simulink model "JCA_LC_Network_Simulation_0p05_Lambda_In_211003"  (R2020a)
settings: Solver=ode15s  StartTime=0.0  StopTime=100*Td  MaxStep=Td/1000  RelTol=1e-3  EnableMultiTasking=on
PreLoadFcn:
  | load gauss_fir;  % pulse shaping coefficients
InitFcn:
  | Zo   =   50;                 %  Line Impedance
  | 
  | Td   =   1/10e6;              % Sinewave period
  | 
  | Ts   =    Td/50     % set this to control simulation speed
  |                           % for wave visualization
  | Tg   =    Td/500;
  | 
  | N=50;                           % secondary to primary turns ratio
  | Cpl_dB=-20*log10(N);    % Coupler coupling coefficent (dB)
libraries: fl_lib x28, nesl_utility x11, simulink x3, ee_lib x2
settings Model: Creator=Dick  LastModifiedBy=Jeff
settings DataIOCC: LimitDataPoints=on  SaveFormat=Array  ReturnWorkspaceOutputs=off
settings OptimizationCC: LifeSpan=inf
settings DebuggingCC: SolverPrmCheckMsg=warning  SFUnexpectedBacktrackingDiag=warning  SFNoUnconditionalDefaultTransitionDiag=warning  SFExecutionAtInitializationDiag=none  ArithmeticOperatorsInVariantConditions=warning
settings HardwareCC: ProdBitPerPointer=32  ProdBitPerSizeT=32  ProdBitPerPtrDiffT=32  ProdLargestAtomicFloat=None  ProdIntDivRoundTo=Undefined  ProdEndianess=Unspecified  ProdWordSize=32  ProdHWDeviceType=32-bit Generic
settings ModelReferenceCC: PropagateSignalLabelsOutOfModel=off
settings SFSimCC: SimUseLocalCustomCode=off  CustomCodeUndefinedFunction=UseInterfaceOnly
settings RTWCC: RTWUseLocalCustomCode=off
settings CodeAppCC: StateflowObjectComments=on
settings GRTTargetCC: TargetLangStandard=C89/C90 (ANSI)
settings ConfigComp: CovMetricSettings=dw  CovHtmlReporting=on  CovSaveCumulativeToWorkspaceVar=on  CovSaveSingleToWorkspaceVar=on  CovExternalEMLEnable=off  CovSFcnEnable=off
settings SimscapeCC: SimscapeNormalizeSystem=off

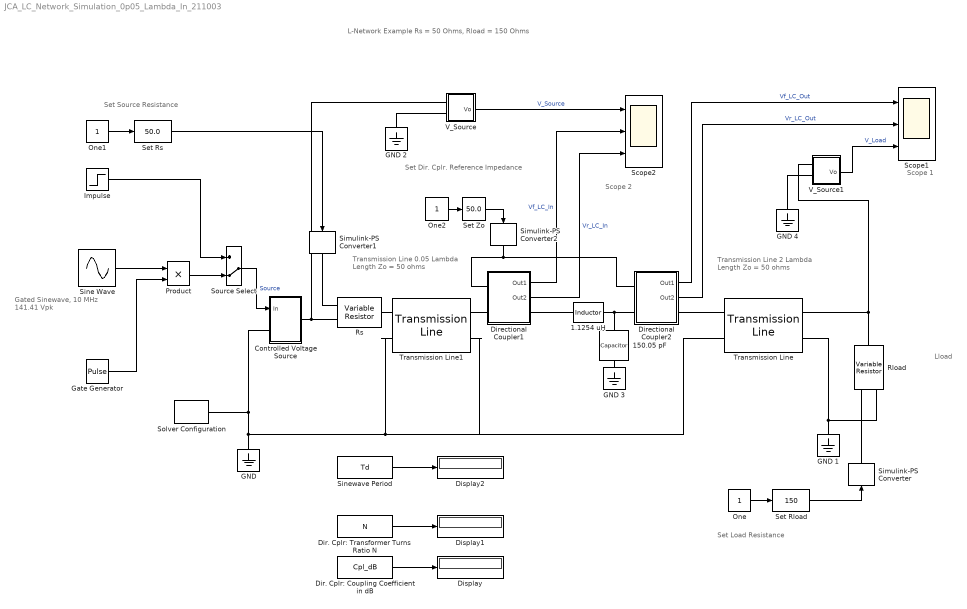
== system JCA_LC_Network_Simulation_0p05_Lambda_In_211003 ==
  note: Lload
  note: Scope 1
  note: L-Network Example
      | Rs = 50 Ohms, Rload = 150 Ohms
  note: Set Load Resistance
  note: Set Source Resistance
  note: Set Dir. Cplr.
      | Reference Impedance
  note: Gated Sinewave,
      | 10 MHz
      | 141.41 Vpk
  note: Transmission Line
      | 2 Lambda Length
      | Zo = 50 ohms
  note: Transmission Line
      | 0.05 Lambda Length
      | Zo = 50 ohms
  note: Scope 2
  1.1254 uH : fl_lib/Electrical/Electrical Elements/Inductor  l=1.1254 uH  r=0 Ohm  g=1e-9 1/Ohm  i_specify=off  i_priority=None  i=0 A  i_nominal_specify=off  i_nominal_unit=A  i_nominal_value=1  v_specify=off  v_priority=None  v=0 V  v_nominal_specify=off  v_nominal_unit=V  v_nominal_value=1  i_L_specify=off  i_L_priority=High  i_L=0 A  i_L_nominal_specify=off  i_L_nominal_unit=A  i_L_nominal_value=1
  150.05 pF : fl_lib/Electrical/Electrical Elements/Capacitor  c=150.05 pF  r=1e-6 Ohm  g=0 1/Ohm  i_specify=off  i_priority=None  i=0 A  i_nominal_specify=off  i_nominal_unit=A  i_nominal_value=1  v_specify=off  v_priority=None  v=0 V  v_nominal_specify=off  v_nominal_unit=V  v_nominal_value=1  vc_specify=off  vc_priority=High  vc=0 V  vc_nominal_specify=off  vc_nominal_unit=V  vc_nominal_value=1
  Controlled Voltage Source : Subsystem
  Dir. Cplr: Coupling Coefficient in dB : Constant  Value=Cpl_dB
  Dir. Cplr: Transformer Turns Ratio N : Constant  Value=N
  Directional Coupler1 : Subsystem
  Directional Coupler2 : Subsystem
  Display : Display
  Display1 : Display
  Display2 : Display
  GND {,1..4} (5 alike) : fl_lib/Electrical/Electrical Elements/Electrical Reference
  Gate Generator : DiscretePulseGenerator  PulseType=Time based  Period=100*Td  PulseWidth=50
  Impulse : Step  Time=Td/1e6  Before=1e13  After=0  SampleTime=0
  One : Constant
  One1 : Constant
  One2 : Constant
  Product : Product
  Rload : fl_lib/Electrical/Electrical Elements/Variable Resistor  Rmin=0 Ohm  i_specify=off  i_priority=High  i=0 A  i_nominal_specify=off  i_nominal_unit=A  i_nominal_value=1  v_specify=off  v_priority=High  v=0 V  v_nominal_specify=off  v_nominal_unit=V  v_nominal_value=1
  Rs : fl_lib/Electrical/Electrical Elements/Variable Resistor  Rmin=0 Ohm  i_specify=off  i_priority=High  i=0 A  i_nominal_specify=off  i_nominal_unit=A  i_nominal_value=1  v_specify=off  v_priority=High  v=0 V  v_nominal_specify=off  v_nominal_unit=V  v_nominal_value=1
  Scope1 : Scope  NumInputPorts=3
  Scope2 : Scope  NumInputPorts=3
  Set Rload : simulink/Math Operations/Slider Gain  gain=150  low=0  high=500
  Set Rs : simulink/Math Operations/Slider Gain  gain=50.0  low=0  high=500
  Set Zo : simulink/Math Operations/Slider Gain  gain=50.0  low=0  high=500
  Simulink-PS Converter : nesl_utility/Simulink-PS Converter  PhysicalDomain=network_engine_domain  SubClassName=ps_input  LeftPortType=input  RightPortType=output  PseudoPeriodic=off  Frequencies=[]  NoiseDistribution=none  NoiseParameters=[]  Unit=1  AffineConversion=off  FilteringAndDerivatives=zero  SimscapeFilterOrder=1  InputFilterTimeConstant=0.001  UdotUserProvided=1
  Simulink-PS Converter1 : nesl_utility/Simulink-PS Converter  PhysicalDomain=network_engine_domain  SubClassName=ps_input  LeftPortType=input  RightPortType=output  PseudoPeriodic=off  Frequencies=[]  NoiseDistribution=none  NoiseParameters=[]  Unit=1  AffineConversion=off  FilteringAndDerivatives=zero  SimscapeFilterOrder=1  InputFilterTimeConstant=0.001  UdotUserProvided=1
  Simulink-PS Converter2 : nesl_utility/Simulink-PS Converter  PhysicalDomain=network_engine_domain  SubClassName=ps_input  LeftPortType=input  RightPortType=output  PseudoPeriodic=off  Frequencies=[]  NoiseDistribution=none  NoiseParameters=[]  Unit=1  AffineConversion=off  FilteringAndDerivatives=zero  SimscapeFilterOrder=1  InputFilterTimeConstant=0.001  UdotUserProvided=1
  Sine Wave : Sin  Amplitude=141.41  Frequency=2*pi/Td  Samples=500  SampleTime=0
  Sinewave Period : Constant  Value=Td
  Solver Configuration : nesl_utility/Solver Configuration  PhysicalDomain=network_engine_domain  SubClassName=solver  LeftPortType=input  RightPortType=generic  Tones=[]  Harmonics=[]  SimulateNoise=off  Profile=off  UseLocalSampling=off  EnableSwitchedLinearOptims=on  FrequencyDomain=off  UseCCode=off  RelTol=0.001  AbsTol=1e-06  MinStep=1e-09  ToWorkspace=off  RevertToSquareIcSolve=off  NumHomotopyIterations=100  PhasorMode=off  PhasorModeNumHarmonics=1  DoDC=off  ResidualTolerance=1e-09  UseLocalSolver=off  LocalSolverChoice=NE_BACKWARD_EULER_ADVANCER  LocalSolverSampleTime=0.001  DoFixedCost=off  MaxNonlinIter=3  MaxModeIter=2  LinearAlgebra=Sparse  EquationFormulation=NE_TIME_EF  DelaysMemoryBudget=1024  AutomaticFiltering=off  FilteringTimeConstant=0.001  PartitionStorageMethod=AS_NEEDED  PartitionMemoryBudget=1024  PartitionMethod=FAST
  Source Select : ManualSwitch  CurrentSetting=0
  Transmission Line : ee_lib/Passive/Lines/Transmission Line  model_type=1  TD=Td*2 s  LC_param=1  Z0_delay_based=50 Ohm  Z0=50 Ohm  freq=60 Hz  Ll=220 uH/m  L=220 uH/m  C=90 pF/m  R=0.3 Ohm/m  G=5e-6 S/m  LEN=1 m  N=1
      settings: SourceProductBaseCode=PS  InternalSimscapePortConfiguration="{\"Bottom\":[],\"Left\":[{\"id\":\"p1\",\"label\":\"\",\"type\":\"foundation.electrical.electrical\"},{\"id\":\"n1\",\"label\":\"\",\"type\":\"foundation.electrical.electrical\"}],\"Right\":[{\"id\":\"p2\",\"label\":\"\",\"type\":\"foundation.electrical.electrical\"},{\"id\":\"n2\",\"label\":\"\",\"type\":\"foundation.electrical.electrical\"}],\"Top\":[]}"
  Transmission Line1 : ee_lib/Passive/Lines/Transmission Line  model_type=1  TD=Td*0.05 s  LC_param=1  Z0_delay_based=50 Ohm  Z0=50 Ohm  freq=60 Hz  Ll=220 uH/m  L=220 uH/m  C=90 pF/m  R=0.3 Ohm/m  G=5e-6 S/m  LEN=1 m  N=1
      settings: SourceProductBaseCode=PS  InternalSimscapePortConfiguration="{\"Bottom\":[],\"Left\":[{\"id\":\"p1\",\"label\":\"\",\"type\":\"foundation.electrical.electrical\"},{\"id\":\"n1\",\"label\":\"\",\"type\":\"foundation.electrical.electrical\"}],\"Right\":[{\"id\":\"p2\",\"label\":\"\",\"type\":\"foundation.electrical.electrical\"},{\"id\":\"n2\",\"label\":\"\",\"type\":\"foundation.electrical.electrical\"}],\"Top\":[]}"
  V_Source : Subsystem
  V_Source1 : Subsystem
  wires:
  Source Select/1 -> Controlled Voltage Source/1(In)  "Source"
  One/1 -> Set Rload/1
  Set Rs/1 -> Simulink-PS Converter1/1
  One1/1 -> Set Rs/1
  Dir. Cplr: Coupling Coefficient in dB/1 -> Display/1
  Dir. Cplr: Transformer Turns Ratio N/1 -> Display1/1
  Sinewave Period/1 -> Display2/1
  One2/1 -> Set Zo/1
  Set Zo/1 -> Simulink-PS Converter2/1
  Product/1 -> Source Select/2
  Sine Wave/1 -> Product/1
  Gate Generator/1 -> Product/2
  Impulse/1 -> Source Select/1
  Set Rload/1 -> Simulink-PS Converter/1
  Directional Coupler2/1(Out1) -> Scope1/1  "Vf_LC_Out"
  Directional Coupler2/2(Out2) -> Scope1/2  "Vr_LC_Out"
  V_Source/1(Vo) -> Scope2/1  "V_Source"
  Directional Coupler1/1(Out1) -> Scope2/2  "Vf_LC_In"
  Directional Coupler1/2(Out2) -> Scope2/3  "Vr_LC_In"
  V_Source1/1(Vo) -> Scope1/3  "V_Load"
  connections:
  Controlled Voltage Source/RConn1 -- Rs/LConn2 -- V_Source/LConn1
  Simulink-PS Converter/RConn1 -- Rload/LConn1
  Simulink-PS Converter1/RConn1 -- Rs/LConn1
  Directional Coupler2/LConn1 -- Directional Coupler1/LConn1 -- Simulink-PS Converter2/RConn1
  Transmission Line/RConn1 -- V_Source1/LConn1 -- Rload/RConn1
  Solver Configuration/RConn1 -- Transmission Line1/RConn2 -- Transmission Line/LConn2 -- Transmission Line1/LConn2 -- "GND "/LConn1 -- Controlled Voltage Source/LConn1
  GND 1/LConn1 -- Rload/LConn2 -- Transmission Line/RConn2
  V_Source/LConn2 -- GND 2/LConn1
  Directional Coupler2/RConn1 -- Transmission Line/LConn1
  1.1254 uH/LConn1 -- Directional Coupler1/RConn1
  V_Source1/LConn2 -- GND 4/LConn1
  GND 3/LConn1 -- 150.05 pF/RConn1
  1.1254 uH/RConn1 -- 150.05 pF/LConn1 -- Directional Coupler2/LConn2
  Transmission Line1/LConn1 -- Rs/RConn1
  Transmission Line1/RConn1 -- Directional Coupler1/LConn2

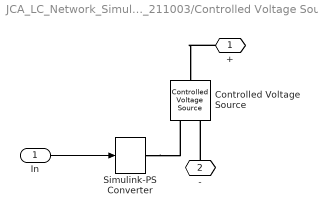
== system JCA_LC_Network_Simulation_0p05_Lambda_In_211003/Controlled Voltage Source ==
  In : Inport
  Controlled Voltage Source : fl_lib/Electrical/Electrical Sources/Controlled Voltage Source
  Simulink-PS Converter : nesl_utility/Simulink-PS Converter  PhysicalDomain=network_engine_domain  SubClassName=ps_input  LeftPortType=input  RightPortType=output  PseudoPeriodic=off  Frequencies=[]  NoiseDistribution=none  NoiseParameters=[]  Unit=1  AffineConversion=off  FilteringAndDerivatives=zero  SimscapeFilterOrder=1  InputFilterTimeConstant=0.001  UdotUserProvided=1
  + : PMIOPort  Side=Right
  - : PMIOPort  Port=2  Side=Left
  wires:
  In/1 -> Simulink-PS Converter/1
  connections:
  +/RConn1 -- Controlled Voltage Source/LConn1
  -/RConn1 -- Controlled Voltage Source/RConn2
  Simulink-PS Converter/RConn1 -- Controlled Voltage Source/RConn1

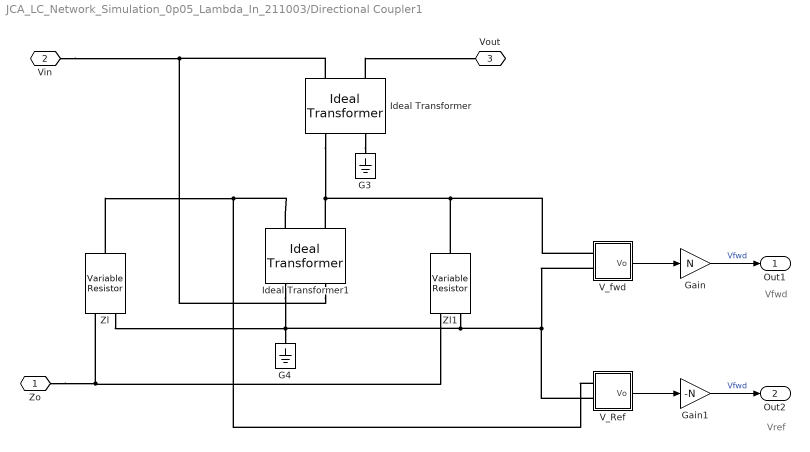
== system JCA_LC_Network_Simulation_0p05_Lambda_In_211003/Directional Coupler1 ==
  note: Vref
  note: Vfwd
  G3 : fl_lib/Electrical/Electrical Elements/Electrical Reference
  G4 : fl_lib/Electrical/Electrical Elements/Electrical Reference
  Gain : Gain  Gain=N
  Gain1 : Gain  Gain=-N
  Ideal Transformer : fl_lib/Electrical/Electrical Elements/Ideal Transformer  n=N  i1_specify=off  i1_priority=None  i1=0 A  i1_nominal_specify=off  i1_nominal_unit=A  i1_nominal_value=1  v1_specify=off  v1_priority=None  v1=0 V  v1_nominal_specify=off  v1_nominal_unit=V  v1_nominal_value=1  i2_specify=off  i2_priority=None  i2=0 A  i2_nominal_specify=off  i2_nominal_unit=A  i2_nominal_value=1  v2_specify=off  v2_priority=None  v2=0 V  v2_nominal_specify=off  v2_nominal_unit=V  v2_nominal_value=1
      settings: AttributesFormatString=%<Name>  SourceProductBaseCode=SS
  Ideal Transformer1 : fl_lib/Electrical/Electrical Elements/Ideal Transformer  n=N  i1_specify=off  i1_priority=None  i1=0 A  i1_nominal_specify=off  i1_nominal_unit=A  i1_nominal_value=1  v1_specify=off  v1_priority=None  v1=0 V  v1_nominal_specify=off  v1_nominal_unit=V  v1_nominal_value=1  i2_specify=off  i2_priority=None  i2=0 A  i2_nominal_specify=off  i2_nominal_unit=A  i2_nominal_value=1  v2_specify=off  v2_priority=None  v2=0 V  v2_nominal_specify=off  v2_nominal_unit=V  v2_nominal_value=1
      settings: AttributesFormatString=%<Name>  SourceProductBaseCode=SS
  V_Ref : Subsystem
  V_fwd : Subsystem
  Zl : fl_lib/Electrical/Electrical Elements/Variable Resistor  Rmin=0 Ohm  i_specify=off  i_priority=High  i=0 A  i_nominal_specify=off  i_nominal_unit=A  i_nominal_value=1  v_specify=off  v_priority=High  v=0 V  v_nominal_specify=off  v_nominal_unit=V  v_nominal_value=1
  Zl1 : fl_lib/Electrical/Electrical Elements/Variable Resistor  Rmin=0 Ohm  i_specify=off  i_priority=High  i=0 A  i_nominal_specify=off  i_nominal_unit=A  i_nominal_value=1  v_specify=off  v_priority=High  v=0 V  v_nominal_specify=off  v_nominal_unit=V  v_nominal_value=1
  Zo : PMIOPort  Side=Left
  Vin : PMIOPort  Port=2  Side=Left
  Vout : PMIOPort  Port=3  Side=Right
  Out1 : Outport
  Out2 : Outport  Port=2
  wires:
  V_fwd/1(Vo) -> Gain/1
  Gain/1 -> Out1/1  "Vfwd"
  Gain1/1 -> Out2/1  "Vfwd"
  V_Ref/1(Vo) -> Gain1/1
  connections:
  Ideal Transformer/LConn1 -- Zl1/RConn1 -- V_fwd/LConn1 -- Ideal Transformer1/RConn2
  Ideal Transformer/RConn1 -- Vin/RConn1 -- Ideal Transformer1/LConn2
  Ideal Transformer1/LConn1 -- V_Ref/LConn2 -- V_fwd/LConn2 -- Zl1/LConn2 -- G4/LConn1 -- Zl/LConn2
  Zl/RConn1 -- Ideal Transformer1/RConn1 -- V_Ref/LConn1
  Ideal Transformer/LConn2 -- G3/LConn1
  Ideal Transformer/RConn2 -- Vout/RConn1
  Zo/RConn1 -- Zl/LConn1 -- Zl1/LConn1

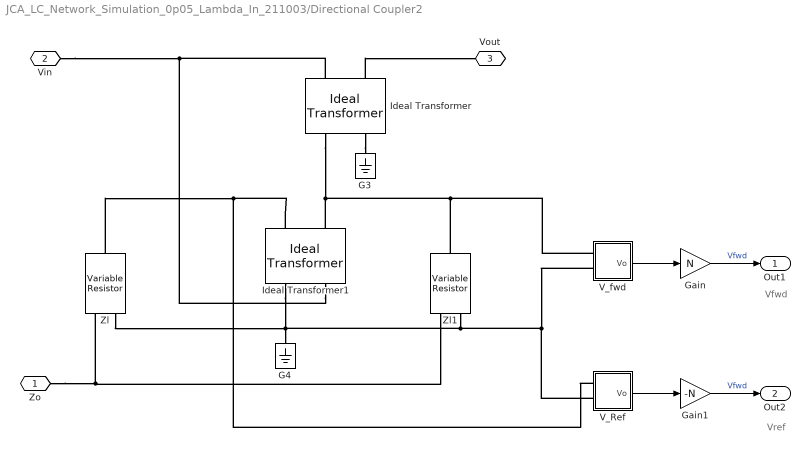
== system JCA_LC_Network_Simulation_0p05_Lambda_In_211003/Directional Coupler2 ==
  note: Vref
  note: Vfwd
  G3 : fl_lib/Electrical/Electrical Elements/Electrical Reference
  G4 : fl_lib/Electrical/Electrical Elements/Electrical Reference
  Gain : Gain  Gain=N
  Gain1 : Gain  Gain=-N
  Ideal Transformer : fl_lib/Electrical/Electrical Elements/Ideal Transformer  n=N  i1_specify=off  i1_priority=None  i1=0 A  i1_nominal_specify=off  i1_nominal_unit=A  i1_nominal_value=1  v1_specify=off  v1_priority=None  v1=0 V  v1_nominal_specify=off  v1_nominal_unit=V  v1_nominal_value=1  i2_specify=off  i2_priority=None  i2=0 A  i2_nominal_specify=off  i2_nominal_unit=A  i2_nominal_value=1  v2_specify=off  v2_priority=None  v2=0 V  v2_nominal_specify=off  v2_nominal_unit=V  v2_nominal_value=1
      settings: AttributesFormatString=%<Name>  SourceProductBaseCode=SS
  Ideal Transformer1 : fl_lib/Electrical/Electrical Elements/Ideal Transformer  n=N  i1_specify=off  i1_priority=None  i1=0 A  i1_nominal_specify=off  i1_nominal_unit=A  i1_nominal_value=1  v1_specify=off  v1_priority=None  v1=0 V  v1_nominal_specify=off  v1_nominal_unit=V  v1_nominal_value=1  i2_specify=off  i2_priority=None  i2=0 A  i2_nominal_specify=off  i2_nominal_unit=A  i2_nominal_value=1  v2_specify=off  v2_priority=None  v2=0 V  v2_nominal_specify=off  v2_nominal_unit=V  v2_nominal_value=1
      settings: AttributesFormatString=%<Name>  SourceProductBaseCode=SS
  V_Ref : Subsystem
  V_fwd : Subsystem
  Zl : fl_lib/Electrical/Electrical Elements/Variable Resistor  Rmin=0 Ohm  i_specify=off  i_priority=High  i=0 A  i_nominal_specify=off  i_nominal_unit=A  i_nominal_value=1  v_specify=off  v_priority=High  v=0 V  v_nominal_specify=off  v_nominal_unit=V  v_nominal_value=1
  Zl1 : fl_lib/Electrical/Electrical Elements/Variable Resistor  Rmin=0 Ohm  i_specify=off  i_priority=High  i=0 A  i_nominal_specify=off  i_nominal_unit=A  i_nominal_value=1  v_specify=off  v_priority=High  v=0 V  v_nominal_specify=off  v_nominal_unit=V  v_nominal_value=1
  Zo : PMIOPort  Side=Left
  Vin : PMIOPort  Port=2  Side=Left
  Vout : PMIOPort  Port=3  Side=Right
  Out1 : Outport
  Out2 : Outport  Port=2
  wires:
  V_fwd/1(Vo) -> Gain/1
  Gain/1 -> Out1/1  "Vfwd"
  Gain1/1 -> Out2/1  "Vfwd"
  V_Ref/1(Vo) -> Gain1/1
  connections:
  Ideal Transformer/LConn1 -- Zl1/RConn1 -- V_fwd/LConn1 -- Ideal Transformer1/RConn2
  Ideal Transformer/RConn1 -- Vin/RConn1 -- Ideal Transformer1/LConn2
  Ideal Transformer1/LConn1 -- V_Ref/LConn2 -- V_fwd/LConn2 -- Zl1/LConn2 -- G4/LConn1 -- Zl/LConn2
  Zl/RConn1 -- Ideal Transformer1/RConn1 -- V_Ref/LConn1
  Ideal Transformer/LConn2 -- G3/LConn1
  Ideal Transformer/RConn2 -- Vout/RConn1
  Zo/RConn1 -- Zl/LConn1 -- Zl1/LConn1

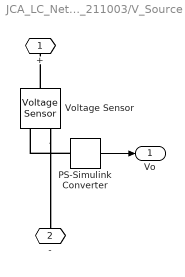
== system JCA_LC_Network_Simulation_0p05_Lambda_In_211003/V_Source ==
  PS-Simulink Converter : nesl_utility/PS-Simulink Converter  PhysicalDomain=network_engine_domain  SubClassName=ps_output  LeftPortType=input  RightPortType=output  PseudoPeriodic=off  Frequencies=[]  Unit=1  AffineConversion=off
  Voltage Sensor : fl_lib/Electrical/Electrical Sensors/Voltage Sensor
  + : PMIOPort  Side=Left
  - : PMIOPort  Port=2  Side=Left
  Vo : Outport
  wires:
  PS-Simulink Converter/1 -> Vo/1
  connections:
  Voltage Sensor/LConn1 -- +/RConn1
  Voltage Sensor/RConn2 -- -/RConn1
  PS-Simulink Converter/LConn1 -- Voltage Sensor/RConn1

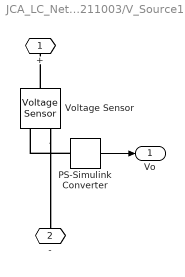
== system JCA_LC_Network_Simulation_0p05_Lambda_In_211003/V_Source1 ==
  PS-Simulink Converter : nesl_utility/PS-Simulink Converter  PhysicalDomain=network_engine_domain  SubClassName=ps_output  LeftPortType=input  RightPortType=output  PseudoPeriodic=off  Frequencies=[]  Unit=1  AffineConversion=off
  Voltage Sensor : fl_lib/Electrical/Electrical Sensors/Voltage Sensor
  + : PMIOPort  Side=Left
  - : PMIOPort  Port=2  Side=Left
  Vo : Outport
  wires:
  PS-Simulink Converter/1 -> Vo/1
  connections:
  Voltage Sensor/LConn1 -- +/RConn1
  Voltage Sensor/RConn2 -- -/RConn1
  PS-Simulink Converter/LConn1 -- Voltage Sensor/RConn1

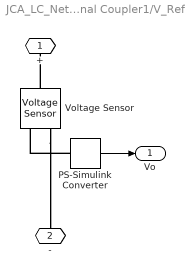
== system JCA_LC_Network_Simulation_0p05_Lambda_In_211003/Directional Coupler1/V_Ref ==
  PS-Simulink Converter : nesl_utility/PS-Simulink Converter  PhysicalDomain=network_engine_domain  SubClassName=ps_output  LeftPortType=input  RightPortType=output  PseudoPeriodic=off  Frequencies=[]  Unit=1  AffineConversion=off
  Voltage Sensor : fl_lib/Electrical/Electrical Sensors/Voltage Sensor
  + : PMIOPort  Side=Left
  - : PMIOPort  Port=2  Side=Left
  Vo : Outport
  wires:
  PS-Simulink Converter/1 -> Vo/1
  connections:
  Voltage Sensor/LConn1 -- +/RConn1
  Voltage Sensor/RConn2 -- -/RConn1
  PS-Simulink Converter/LConn1 -- Voltage Sensor/RConn1

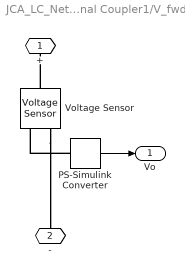
== system JCA_LC_Network_Simulation_0p05_Lambda_In_211003/Directional Coupler1/V_fwd ==
  PS-Simulink Converter : nesl_utility/PS-Simulink Converter  PhysicalDomain=network_engine_domain  SubClassName=ps_output  LeftPortType=input  RightPortType=output  PseudoPeriodic=off  Frequencies=[]  Unit=1  AffineConversion=off
  Voltage Sensor : fl_lib/Electrical/Electrical Sensors/Voltage Sensor
  + : PMIOPort  Side=Left
  - : PMIOPort  Port=2  Side=Left
  Vo : Outport
  wires:
  PS-Simulink Converter/1 -> Vo/1
  connections:
  Voltage Sensor/LConn1 -- +/RConn1
  Voltage Sensor/RConn2 -- -/RConn1
  PS-Simulink Converter/LConn1 -- Voltage Sensor/RConn1

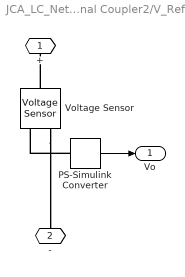
== system JCA_LC_Network_Simulation_0p05_Lambda_In_211003/Directional Coupler2/V_Ref ==
  PS-Simulink Converter : nesl_utility/PS-Simulink Converter  PhysicalDomain=network_engine_domain  SubClassName=ps_output  LeftPortType=input  RightPortType=output  PseudoPeriodic=off  Frequencies=[]  Unit=1  AffineConversion=off
  Voltage Sensor : fl_lib/Electrical/Electrical Sensors/Voltage Sensor
  + : PMIOPort  Side=Left
  - : PMIOPort  Port=2  Side=Left
  Vo : Outport
  wires:
  PS-Simulink Converter/1 -> Vo/1
  connections:
  Voltage Sensor/LConn1 -- +/RConn1
  Voltage Sensor/RConn2 -- -/RConn1
  PS-Simulink Converter/LConn1 -- Voltage Sensor/RConn1

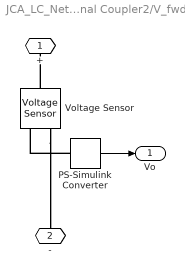
== system JCA_LC_Network_Simulation_0p05_Lambda_In_211003/Directional Coupler2/V_fwd ==
  PS-Simulink Converter : nesl_utility/PS-Simulink Converter  PhysicalDomain=network_engine_domain  SubClassName=ps_output  LeftPortType=input  RightPortType=output  PseudoPeriodic=off  Frequencies=[]  Unit=1  AffineConversion=off
  Voltage Sensor : fl_lib/Electrical/Electrical Sensors/Voltage Sensor
  + : PMIOPort  Side=Left
  - : PMIOPort  Port=2  Side=Left
  Vo : Outport
  wires:
  PS-Simulink Converter/1 -> Vo/1
  connections:
  Voltage Sensor/LConn1 -- +/RConn1
  Voltage Sensor/RConn2 -- -/RConn1
  PS-Simulink Converter/LConn1 -- Voltage Sensor/RConn1
